simulink model "myrobot_controller"  (R2023b)
settings: Solver=VariableStepAuto  StartTime=0.0  StopTime=25  RelTol=1e-3
settings Model: Creator=duong  LastModifiedBy=Admin
settings DebuggingCC: UnconnectedInputMsg=warning  UnconnectedOutputMsg=warning  UnconnectedLineMsg=warning
settings ModelReferenceCC: EnableRefExpFcnMdlSchedulingChecks=on
settings RTWCC: DLArmComputeVersion=19.05

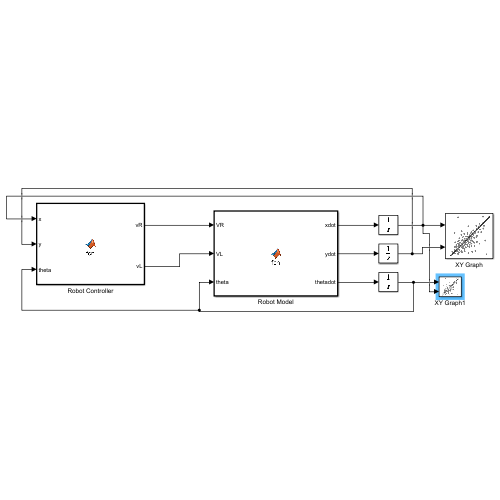
[thumbnail: Simulink's stored preview of the top-level diagram]
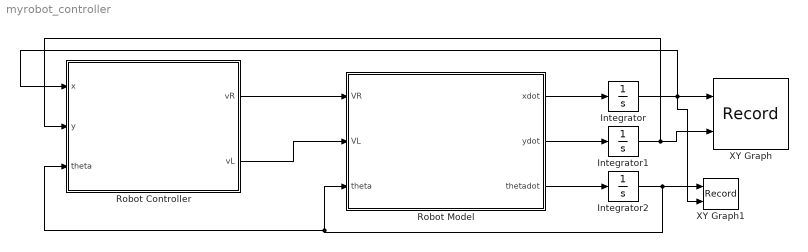
== system myrobot_controller ==
  Integrator : Integrator
  Integrator1 : Integrator
  Integrator2 : Integrator
  Robot Controller : MATLAB Function  TreatAsAtomicUnit=on
  Robot Model : MATLAB Function  TreatAsAtomicUnit=on
  XY Graph : Record  FileSettingsInternal="{\"entries\":[{\"content\":{\"excelSettings\":{\"content\":{},\"type\":\"Streamout.ExcelSettings\"}},\"type\":\"Streamout.FileSettingStorage\",\"uuid\":\"\"}],\"packageUris\":[\"http:\\/\\/schema.mathworks.com\\/mf0\\/streamout_blocks\\/R2020a\"],\"version\":\"1.0\"}"  Layout=[1 1]  SignalsInternal="{\"entries\":[{\"content\":{\"signals\":[{\"content\":{\"blockPath\":[],\"dimensions\":[1],\"domain\":\"\",\"lineColor\":\"#a2142f\",\"plots\":[1],\"port\":1,\"sid\":[\"\"],\"signalID\":120,\"signalName\":\"Integrator\"},\"type\":\"RecordBlkView.Signal\",\"uuid\":\"\"},{\"content\":{\"blockPath\":[],\"dimensions\":[1],\"domain\":\"\",\"lineColor\":\"#139fff\",\"plots\":[1],\"port\":2,\"sid\":[\"\"],\"signalID\":124,\"signalName\":\"Integrator1\"},\"type\":\"RecordBlkView.Signal\",\"uuid\":\"\"}]},\"type\":\"RecordBlkView.InputSignals\",\"uuid\":\"\"}],\"packageUris\":[\"http:\\/\\/schema.mathworks.com\\/mf0\\/streamout_blocks\\/R2020a\"],\"version\":\"1.0\"}"  VisualizationBindings="{\"xyplotplugin\":{\"info\":[{\"series\":[{\"bindingParametersList\":[{\"parameter\":\"X-Axis\",\"signalID\":120,\"signalName\":\"Integrator\"},{\"parameter\":\"Y-Axis\",\"signalID\":124,\"signalName\":\"Integrator1\"}],\"seriesID\":33293}],\"subplotID\":1}]}}"  CompatibilityTag=XY  st=-1
  XY Graph1 : Record  FileSettingsInternal="{\"entries\":[{\"content\":{\"excelSettings\":{\"content\":{},\"type\":\"Streamout.ExcelSettings\"}},\"type\":\"Streamout.FileSettingStorage\",\"uuid\":\"\"}],\"packageUris\":[\"http:\\/\\/schema.mathworks.com\\/mf0\\/streamout_blocks\\/R2020a\"],\"version\":\"1.0\"}"  Layout=[1 1]  SignalsInternal="{\"entries\":[{\"content\":{\"signals\":[{\"content\":{\"blockPath\":[],\"dimensions\":[1],\"domain\":\"\",\"lineColor\":\"#a2142f\",\"plots\":[1],\"port\":1,\"sid\":[\"\"],\"signalID\":128,\"signalName\":\"Integrator2\"},\"type\":\"RecordBlkView.Signal\",\"uuid\":\"\"},{\"content\":{\"blockPath\":[],\"dimensions\":[1],\"domain\":\"\",\"lineColor\":\"#139fff\",\"plots\":[1],\"port\":2,\"sid\":[\"\"],\"signalID\":132,\"signalName\":\"Integrator\"},\"type\":\"RecordBlkView.Signal\",\"uuid\":\"\"}]},\"type\":\"RecordBlkView.InputSignals\",\"uuid\":\"\"}],\"packageUris\":[\"http:\\/\\/schema.mathworks.com\\/mf0\\/streamout_blocks\\/R2020a\"],\"version\":\"1.0\"}"  VisualizationBindings="{\"xyplotplugin\":{\"info\":[{\"series\":[{\"bindingParametersList\":[{\"parameter\":\"X-Axis\",\"signalID\":128,\"signalName\":\"Integrator2\"},{\"parameter\":\"Y-Axis\",\"signalID\":132,\"signalName\":\"Integrator\"}],\"seriesID\":10115}],\"subplotID\":1}]}}"  CompatibilityTag=XY
  wires:
  Robot Model/3(thetadot) -> Integrator2/1
  Integrator2/1 -> XY Graph1/1, Robot Controller/3(theta), Robot Model/3(theta)
  Robot Model/1(xdot) -> Integrator/1
  Robot Model/2(ydot) -> Integrator1/1
  Integrator/1 -> XY Graph1/2, XY Graph/1, Robot Controller/1(x)
  Integrator1/1 -> Robot Controller/2(y), XY Graph/2
  Robot Controller/1(vR) -> Robot Model/1(VR)
  Robot Controller/2(vL) -> Robot Model/2(VL)

== matlab function myrobot_controller/Robot Controller ==
  data: vR output; x input; vL output; y input; theta input
function [vR,vL] = fcn(x, y, theta)
target = [5 5 0];

% Control parameters
gamma=3;
lamda=1000;
h=2;

% Robot parameter: Distance between two wheels
d=0.5;

% Calculate polar variables
rho = sqrt((target(1)-x)^2+(target(2)-y)^2);
phi = atan2(target(2)-y,target(1)-x)-target(3);
alpha = phi+target(3)-theta;

% Calculate control laws
v = gamma*cos(alpha)*rho;
w = lamda*alpha + gamma*cos(alpha)*sin(alpha)/alpha*(alpha+h*phi);

% Calculate Vl and Vr from v and w
vL = (2*v-d*w)/2;
vR = (2*v+d*w)/2;

== matlab function myrobot_controller/Robot Model ==
  data: VR input; xdot output; VL input; theta input; ydot output; thetadot output
function [xdot, ydot, thetadot] = fcn(VR, VL,theta)

l=0.18; % distance between 2 driven wheels
xdot=(VR+VL)/2*cos(theta);
ydot=(VR+VL)/2*sin(theta);
thetadot=(VR-VL)/l;
